simulink model "System_TargetTracking_PF_Simulation"  (Simulink 6.3)
settings: Solver=VariableStepDiscrete  StartTime=0.0  StopTime=40.0  RelTol=1e-3
libraries: simulink x2
settings Model: LastModifiedBy=Huang

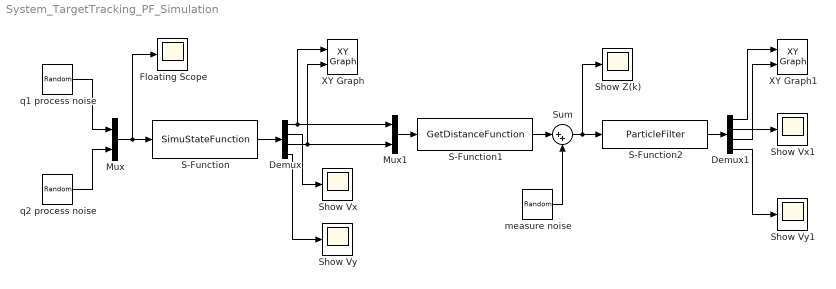
== system System_TargetTracking_PF_Simulation ==
  Demux : Demux
  Demux1 : Demux
  Floating Scope : Scope
      settings: TimeRange=10  YMin=-3  YMax=2
  Mux : Mux  Description=Mux  Inputs=2
  Mux1 : Mux  Inputs=2
  S-Function : S-Function  FunctionName=SimuStateFunction
  S-Function1 : S-Function  FunctionName=GetDistanceFunction
  S-Function2 : S-Function  FunctionName=ParticleFilter
  Show Vx : Scope
      settings: YMin=1  YMax=6
  Show Vx1 : Scope
      settings: SaveName=ScopeData5
  Show Vy : Scope
      settings: YMin=2  YMax=7  SaveName=ScopeData2
  Show Vy1 : Scope
      settings: SaveName=ScopeData6
  Show Z(k) : Scope
      settings: SaveName=ScopeData3
  Sum : Sum  Inputs=|++
  XY Graph : simulink/Sinks/XY Graph  xmin=0  xmax=600  ymin=0  ymax=600  st=1
  XY Graph1 : simulink/Sinks/XY Graph  xmin=0  xmax=600  ymin=0  ymax=600  st=1
  measure noise : RandomNumber  Variance=0.01  SampleTime=1
  q1 process noise : RandomNumber  Variance=0.0001  SampleTime=1
  q2 process noise : RandomNumber  Variance=0.0009  Seed=3  SampleTime=1
  wires:
  q1 process noise/1 -> Mux/1
  q2 process noise/1 -> Mux/2
  Mux/1 -> Floating Scope/1, S-Function/1
  S-Function/1 -> Demux/1
  Demux/1 -> XY Graph/1, Mux1/1
  Demux/3 -> XY Graph/2, Mux1/2
  Demux/4 -> Show Vy/1
  Demux/2 -> Show Vx/1
  Demux1/1 -> XY Graph1/1
  Demux1/3 -> XY Graph1/2
  Demux1/2 -> Show Vx1/1
  Demux1/4 -> Show Vy1/1
  Mux1/1 -> S-Function1/1
  S-Function2/1 -> Demux1/1
  S-Function1/1 -> Sum/1
  measure noise/1 -> Sum/2
  Sum/1 -> S-Function2/1, Show Z(k)/1
